simulink model "sf_pw_switch4_"  (Simulink 7.4)
settings: Solver=ode45  StartTime=0.0  StopTime=10.0  RelTol=1e-3
settings Model: Creator=rcobbe  LastModifiedBy=rcobbe

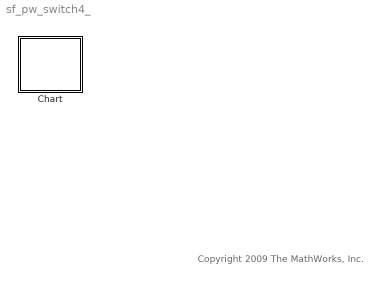
== system sf_pw_switch4_ ==
  note: Copyright 2009 The MathWorks, Inc.
  Chart : Stateflow chart

== stateflow chart Chart ==
  note: Do not put any code along
      | the transitions that run
      | down the right side!
  (junction 12) -> (junction 4) [order 1] : [case1]
  (junction 4) -> (junction 5) : {action1}
  (junction 5) -> (junction 13)
  (junction 13) -> (junction 19)
  (junction 14) -> (junction 7) [order 1] : [case2]
  (junction 7) -> (junction 6) : {action2}
  (junction 6) -> (junction 19)
  (junction 12) -> (junction 14) [order 2]
  (junction 14) -> (junction 15) [order 2]
  (junction 19) -> (junction 20)
  (junction 15) -> (junction 10) [order 1] : [case3]
  (junction 10) -> (junction 11) : {action3}
  (junction 11) -> (junction 20)
  (junction 15) -> (junction 16) [order 2]
  (junction 20) -> (junction 21)
  (junction 16) -> (junction 9) [order 1] : [case4]
  (junction 9) -> (junction 8) : {action4}
  (junction 8) -> (junction 21)
  (junction 16) -> (junction 17) [order 2] : {defaultAction}
  (junction 21) -> (junction 22)
  (junction 17) -> (junction 18)
  (junction 22) -> (junction 17)
  (default) -> (junction 12) : /*comment*/
